simulink library "mergelibrary"  (Simulink 6.6)
settings Model: Creator=hnine  LastModifiedBy=hnine

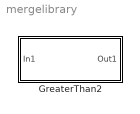
== system mergelibrary ==
  GreaterThan2 : Subsystem

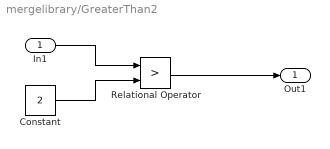
== system mergelibrary/GreaterThan2 ==
  In1 : Inport
  Constant : Constant  Value=2
  Relational Operator : RelationalOperator  Operator=>  LogicOutDataTypeMode=Boolean
  Out1 : Outport
  wires:
  In1/1 -> Relational Operator/1
  Constant/1 -> Relational Operator/2
  Relational Operator/1 -> Out1/1
